simulink model "Final_PAPER2_wtdelay_LQR"  (R2024b)
settings: Solver=ode23  StartTime=0.0  StopTime=6  RelTol=1e-3
undefined symbols (not defined in the file): Q, R, sigbuilder_block
libraries: simulink_extras x4, simulink x1
settings Model: Creator=HP  LastModifiedBy=shree
settings OptimizationCC: ReuseModelBlockBuffer=off
settings RTWCC: GPUComputeCapability=3.5

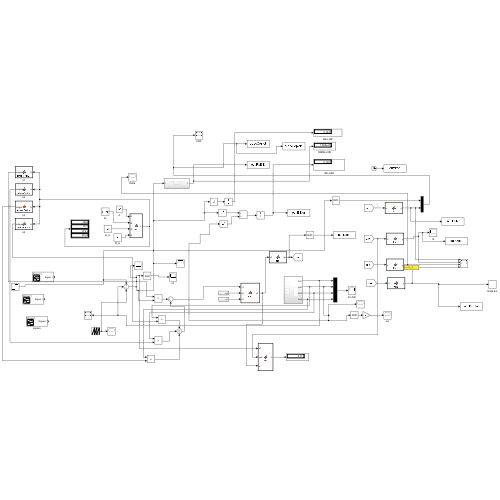
[thumbnail: Simulink's stored preview of the top-level diagram]
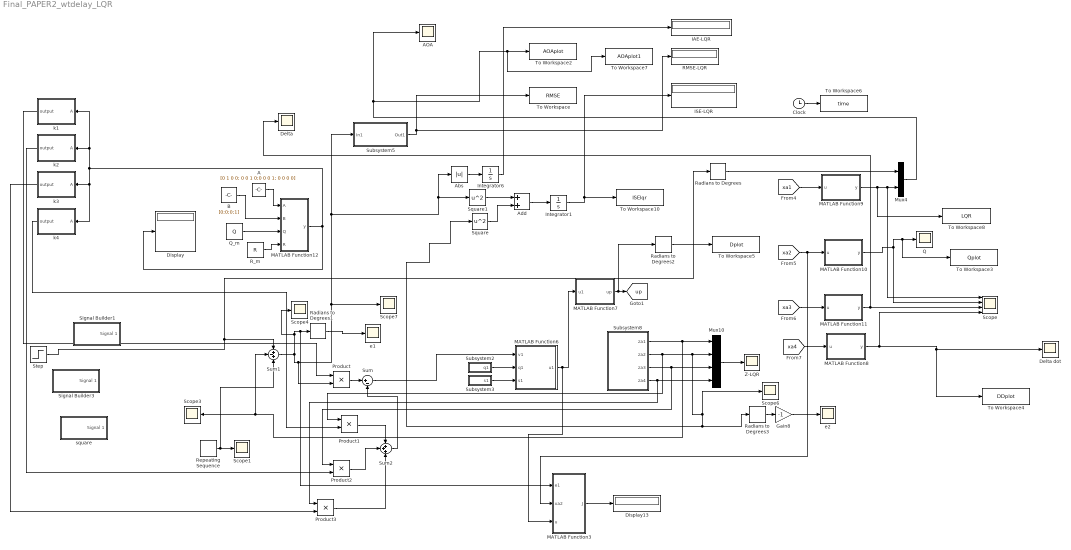
== system Final_PAPER2_wtdelay_LQR ==
  A : Constant  Value=[0 1 0 0; 0 0 1 0;0 0 0 1; 0 0 0 0]
  AOA : Scope
  Abs : Abs  SaturateOnIntegerOverflow=off
  Add : Sum
  B : Constant  Value=[0;0;0;1]
  Clock : Clock
      settings: Decimation=6
  Delta : Scope
  Delta dot : Scope
  Display : Display
  Display13 : Display
  Gain8 : Gain  Gain=-1
  IAE-LQR : Display
  ISE-LQR : Display
  Integrator1 : Integrator
  Integrator6 : Integrator
  MATLAB Function10 : MATLAB Function  TreatAsAtomicUnit=on
  MATLAB Function11 : MATLAB Function  TreatAsAtomicUnit=on
  MATLAB Function12 : MATLAB Function  TreatAsAtomicUnit=on
  MATLAB Function3 : MATLAB Function  TreatAsAtomicUnit=on
  MATLAB Function6 : MATLAB Function  TreatAsAtomicUnit=on
  MATLAB Function7 : MATLAB Function  TreatAsAtomicUnit=on
  MATLAB Function8 : MATLAB Function  TreatAsAtomicUnit=on
  MATLAB Function9 : MATLAB Function  TreatAsAtomicUnit=on
  Mux10 : Mux
  Mux4 : Mux  Inputs=2
  Product{,1..3} (4 alike) : Product
  Q : Scope
  Q_m : Constant  Value=Q
  RMSE-LQR : Display
  R_m : Constant  Value=R
  Radians to Degrees{,1..3} (4 alike) : simulink_extras/Transformations/Radians to Degrees
  Repeating Sequence : simulink/Sources/Repeating Sequence  rep_seq_t=t  rep_seq_y=u_combined
  Scope : Scope  NumInputPorts=4
  Scope{1,3..4,6..7} (5 alike) : Scope
  Signal Builder1 : Subsystem  Tag=STV Subsys  LoadFcn=sigbuilder_block('load');  StartFcn=sigbuilder_block('start');  StopFcn=sigbuilder_block('stop');  ClipboardFcn=sigbuilder_block('clipboard');  mask(Sigbuilder block){tuvar=[0:10]}
      mask help: Simulink:masks:SigbuilderBlock_MD
      mask init:
      | if ~strcmp(get_param(bdroot(gcbh),'SimulationStatus'),'stopped') tuvar = sigbuilder_block('maskInit'); end
      settings: CopyFcn=sigbuilder_block('copy');  DeleteFcn=sigbuilder_block('delete');  ModelCloseFcn=sigbuilder_block('modelClose');  PreSaveFcn=sigbuilder_block('preSave');  PauseFcn=sigbuilder_block('pause');  ContinueFcn=sigbuilder_block('continue');  NameChangeFcn=sigbuilder_block('namechange');  OpenFcn=sigbuilder_block('open',[5.4 -24.6 1141.2 477.6 ]);  CloseFcn=sigbuilder_block('close');
      mask Display: plot(0, 0, 100, 100,[2, 2, 32, 32, 2], [68, 8, 8, 68, 68],[32, 2], [38, 38], [32, 19, 2],[53, 60, 44], [32, 17, 17, 2],[16, 16, 31, 31]);txt = getActiveGroup(gcbh);text(2, 100, txt,'verticalAlignment', 'top');
  Signal Builder3 : Subsystem  Tag=STV Subsys  LoadFcn=sigbuilder_block('load');  StartFcn=sigbuilder_block('start');  StopFcn=sigbuilder_block('stop');  ClipboardFcn=sigbuilder_block('clipboard');  mask(Sigbuilder block){tuvar=[0:10]}
      mask help: Simulink:masks:SigbuilderBlock_MD
      mask init:
      | if ~strcmp(get_param(bdroot(gcbh),'SimulationStatus'),'stopped') tuvar = sigbuilder_block('maskInit'); end
      settings: CopyFcn=sigbuilder_block('copy');  DeleteFcn=sigbuilder_block('delete');  ModelCloseFcn=sigbuilder_block('modelClose');  PreSaveFcn=sigbuilder_block('preSave');  PauseFcn=sigbuilder_block('pause');  ContinueFcn=sigbuilder_block('continue');  NameChangeFcn=sigbuilder_block('namechange');  OpenFcn=sigbuilder_block('open',[5.4 -40.2 1141.2 515.4 ]);  CloseFcn=sigbuilder_block('close');
      mask Display: plot(0, 0, 100, 100,[2, 2, 32, 32, 2], [68, 8, 8, 68, 68],[32, 2], [38, 38], [32, 19, 2],[53, 60, 44], [32, 17, 17, 2],[16, 16, 31, 31]);txt = getActiveGroup(gcbh);text(2, 100, txt,'verticalAlignment', 'top');
  Square : Math  Operator=square
  Square1 : Math  Operator=square
  Step : Step  Time=0  After=0.2617795  SampleTime=0
  Subsystem2 : Subsystem
  Subsystem3 : Subsystem
  Subsystem5 : Subsystem
  Subsystem8 : Subsystem
  Sum : Sum  Inputs=|+-
  Sum1 : Sum  Inputs=+-+
  Sum2 : Sum  Inputs=+++
  To Workspace : ToWorkspace  VariableName=RMSE  SampleTime=-1
  To Workspace10 : ToWorkspace  VariableName=ISElqr  SampleTime=-1
  To Workspace2 : ToWorkspace  VariableName=AOAplot  SampleTime=-1
  To Workspace3 : ToWorkspace  VariableName=Qplot  SaveFormat=Timeseries  SampleTime=-1
  To Workspace4 : ToWorkspace  VariableName=DDplot  SaveFormat=Timeseries  SampleTime=-1
  To Workspace5 : ToWorkspace  VariableName=Dplot  SaveFormat=Timeseries  SampleTime=-1
  To Workspace6 : ToWorkspace  VariableName=time  SaveFormat=Timeseries  SampleTime=-1
  To Workspace7 : ToWorkspace  VariableName=AOAplot1  SampleTime=-1
  To Workspace8 : ToWorkspace  VariableName=LQR  SaveFormat=Timeseries  SampleTime=-1
  Z-LQR : Scope
  e1 : Scope
  e2 : Scope
  k1 : MATLAB Function  TreatAsAtomicUnit=on
  k2 : MATLAB Function  TreatAsAtomicUnit=on
  k3 : MATLAB Function  TreatAsAtomicUnit=on
  k4 : MATLAB Function  TreatAsAtomicUnit=on
  square : Subsystem  Tag=STV Subsys  LoadFcn=sigbuilder_block('load');  StartFcn=sigbuilder_block('start');  StopFcn=sigbuilder_block('stop');  ClipboardFcn=sigbuilder_block('clipboard');  mask(Sigbuilder block){tuvar=[0:10]}
      mask help: Simulink:masks:SigbuilderBlock_MD
      mask init:
      | if ~strcmp(get_param(bdroot(gcbh),'SimulationStatus'),'stopped') tuvar = sigbuilder_block('maskInit'); end
      settings: CopyFcn=sigbuilder_block('copy');  DeleteFcn=sigbuilder_block('delete');  ModelCloseFcn=sigbuilder_block('modelClose');  PreSaveFcn=sigbuilder_block('preSave');  PauseFcn=sigbuilder_block('pause');  ContinueFcn=sigbuilder_block('continue');  NameChangeFcn=sigbuilder_block('namechange');  OpenFcn=sigbuilder_block('open',[5.4 36 1141.2 516.6 ]);  CloseFcn=sigbuilder_block('close');
      mask Display: plot(0, 0, 100, 100,[2, 2, 32, 32, 2], [68, 8, 8, 68, 68],[32, 2], [38, 38], [32, 19, 2],[53, 60, 44], [32, 17, 17, 2],[16, 16, 31, 31]);txt = getActiveGroup(gcbh);text(2, 100, txt,'verticalAlignment', 'top');
  tag scope: up=global
  wires:
  [xa4] -> MATLAB Function8/1(u)
  Subsystem2/1(q1) -> MATLAB Function6/2(q1)
  Subsystem3/1(s1) -> MATLAB Function6/3(s1)
  MATLAB Function6/1(u1) -> MATLAB Function3/3(u), MATLAB Function7/1(u1)
  [xa3] -> MATLAB Function11/1(u)
  [xa2] -> MATLAB Function3/2(xa2), MATLAB Function10/1(u)
  MATLAB Function10/1(y) -> Scope/2, Q/1, To Workspace3/1
  MATLAB Function11/1(y) -> Delta/1, Scope/3
  [xa1] -> MATLAB Function9/1(u)
  Mux4/1 -> AOA/1, To Workspace7/1, To Workspace2/1
  Integrator1/1 -> To Workspace10/1, ISE-LQR/1
  Subsystem5/1(Out1) -> To Workspace/1, RMSE-LQR/1
  Sum1/1 -> Scope4/1, MATLAB Function3/1(e1), Radians to Degrees1/1, Product/2, Scope7/1, Square1/1, Abs/1, Subsystem5/1(In1)
  Abs/1 -> Integrator6/1
  Integrator6/1 -> IAE-LQR/1
  MATLAB Function7/1(up) -> Radians to Degrees2/1, [up]
  Mux10/1 -> Z-LQR/1
  Subsystem8/4(za4) -> Product3/1, Mux10/4
  Subsystem8/3(za3) -> Product2/1, Mux10/3
  Subsystem8/1(za1) -> Sum1/2, Scope3/1, Mux10/1
  MATLAB Function9/1(y) -> To Workspace8/1, Scope/1, Mux4/2
  MATLAB Function8/1(y) -> Scope/4, Delta dot/1, To Workspace4/1
  Radians to Degrees/1 -> Mux4/1
  Clock/1 -> To Workspace6/1
  Radians to Degrees1/1 -> e1/1
  Radians to Degrees2/1 -> To Workspace5/1
  Subsystem8/2(za2) -> Product1/1, Scope6/1, Radians to Degrees3/1, Square/1, Mux10/2
  Radians to Degrees3/1 -> Gain8/1
  Gain8/1 -> e2/1
  Add/1 -> Integrator1/1
  Square/1 -> Add/2
  Square1/1 -> Add/1
  MATLAB Function3/1(J) -> Display13/1
  Sum2/1 -> Sum/2
  Sum/1 -> MATLAB Function6/1(v1)
  Step/1 -> Radians to Degrees/1, Sum1/1
  MATLAB Function12/1(y) -> k1/1(A), k2/1(A), k4/1(A), k3/1(A), Display/1
  B/1 -> MATLAB Function12/2(B)
  A/1 -> MATLAB Function12/1(A)
  k1/1(output) -> Product/1
  Product/1 -> Sum/1
  k4/1(output) -> Product1/2
  Product1/1 -> Sum2/1
  k2/1(output) -> Product2/2
  Product2/1 -> Sum2/2
  k3/1(output) -> Product3/2
  Product3/1 -> Sum2/3
  Q_m/1 -> MATLAB Function12/3(Q)
  R_m/1 -> MATLAB Function12/4(R)
  Repeating Sequence/1 -> Sum1/3, Scope1/1

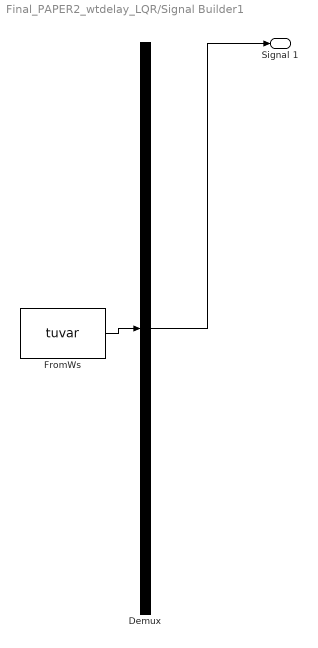
== system Final_PAPER2_wtdelay_LQR/Signal Builder1 ==
  Demux : Demux  Tag=STV Demux  Outputs=1
      settings: DisplayOption=none
  FromWs : FromWorkspace  Tag=STV FromWs  VariableName=tuvar
      SigBuilderData=|
      | common.afterFinalStr = 'Extrapolate'
      | common.sampleTime = 0
      | dataSet.timeRange = [0 10]
      | dataSet.name = 'Group 1'
      | sbobj.Groups.Name = 'Group 1'
      | sbobj.Groups.Signals.Name = 'Signal 1'
      | sbobj.Groups.Signals.XData = [0 2 2 4 4 6 6 8 8 10]
      | sbobj.Groups.Signals.YData = [-0.176 -0.176 0.176 0.176 -0.176 -0.176 0.176 0.176 -0.176 -0.176]
  Signal 1 : Outport  Tag=STV Outport
  wires:
  Demux/1 -> Signal 1/1
  FromWs/1 -> Demux/1

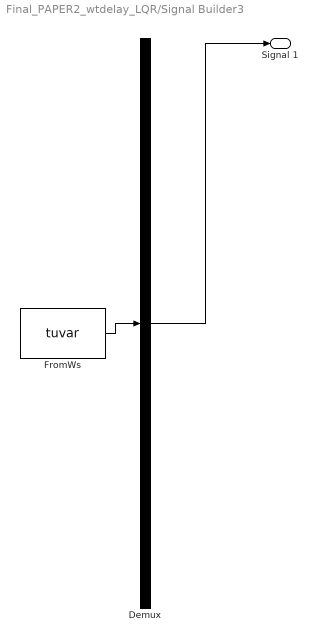
== system Final_PAPER2_wtdelay_LQR/Signal Builder3 ==
  Demux : Demux  Tag=STV Demux  Outputs=1
      settings: DisplayOption=none
  FromWs : FromWorkspace  Tag=STV FromWs  VariableName=tuvar
      SigBuilderData=|
      | common.afterFinalStr = 'Extrapolate'
      | common.sampleTime = 0
      | dataSet.timeRange = [0 6]
      | dataSet.name = 'Group 1'
      | sbobj.Groups.Name = 'Group 1'
      | sbobj.Groups.Signals.Name = 'Signal 1'
      | sbobj.Groups.Signals.XData = [0 2 2 4 4 6]
      | sbobj.Groups.Signals.YData = [0.261799 0.261799 -0.261799 -0.261799 0.261799 0.261799]
      | sbobj.Groups.TimeRange = [0 6]
  Signal 1 : Outport  Tag=STV Outport
  wires:
  Demux/1 -> Signal 1/1
  FromWs/1 -> Demux/1

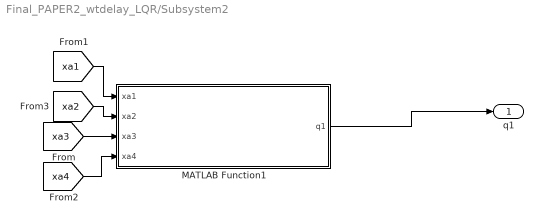
== system Final_PAPER2_wtdelay_LQR/Subsystem2 ==
  MATLAB Function1 : MATLAB Function  TreatAsAtomicUnit=on
  q1 : Outport
  wires:
  [xa2] -> MATLAB Function1/2(xa2)
  [xa1] -> MATLAB Function1/1(xa1)
  MATLAB Function1/1(q1) -> q1/1
  [xa3] -> MATLAB Function1/3(xa3)
  [xa4] -> MATLAB Function1/4(xa4)

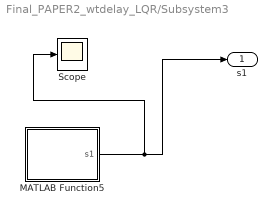
== system Final_PAPER2_wtdelay_LQR/Subsystem3 ==
  MATLAB Function5 : MATLAB Function  TreatAsAtomicUnit=on
  Scope : Scope
  s1 : Outport
  wires:
  MATLAB Function5/1(s1) -> Scope/1, s1/1

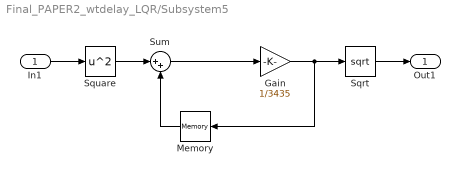
== system Final_PAPER2_wtdelay_LQR/Subsystem5 ==
  In1 : Inport
  Gain : Gain  Gain=1/3435
  Memory : Memory
  Sqrt : Sqrt
  Square : Math  Operator=square
  Sum : Sum  Inputs=|++
  Out1 : Outport
  wires:
  In1/1 -> Square/1
  Square/1 -> Sum/1
  Memory/1 -> Sum/2
  Sum/1 -> Gain/1
  Gain/1 -> Sqrt/1, Memory/1
  Sqrt/1 -> Out1/1

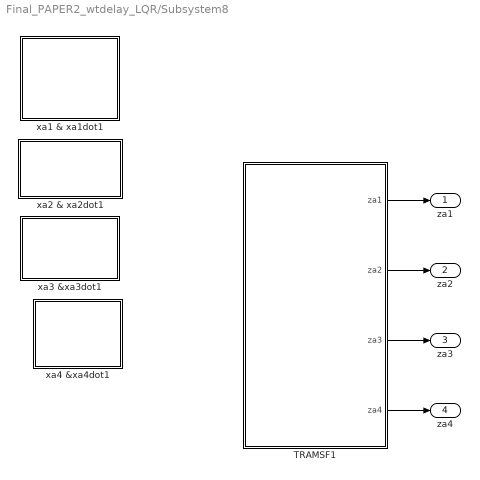
== system Final_PAPER2_wtdelay_LQR/Subsystem8 ==
  " xa3 &xa3dot1" : Subsystem
  TRAMSF1 : Subsystem
  xa1 & xa1dot1 : Subsystem
  xa2 & xa2dot1 : Subsystem
  xa4 &xa4dot1 : Subsystem
  za1 : Outport
  za2 : Outport  Port=2
  za3 : Outport  Port=3
  za4 : Outport  Port=4
  wires:
  TRAMSF1/1(za1) -> za1/1
  TRAMSF1/3(za3) -> za3/1
  TRAMSF1/2(za2) -> za2/1
  TRAMSF1/4(za4) -> za4/1

== system Final_PAPER2_wtdelay_LQR/square ==
  Demux : Demux  Tag=STV Demux  Outputs=1
      settings: DisplayOption=none
  FromWs : FromWorkspace  Tag=STV FromWs  VariableName=tuvar
      SigBuilderData=|
      | common.afterFinalStr = 'Extrapolate'
      | common.sampleTime = 0
      | dataSet.timeRange = [0 10]
      | dataSet.name = 'Group 1'
      | sbobj.Groups.Name = 'Group 1'
      | sbobj.Groups.Signals.Name = 'Signal 1'
      | sbobj.Groups.Signals.XData = [0 2 2 4 4 10]
      | sbobj.Groups.Signals.YData = [0.2617 0.2617 -0.176 -0.176 0.176 0.176]
  Signal 1 : Outport  Tag=STV Outport
  wires:
  Demux/1 -> Signal 1/1
  FromWs/1 -> Demux/1

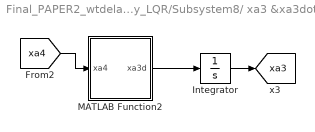
== system Final_PAPER2_wtdelay_LQR/Subsystem8/ xa3 &xa3dot1 ==
  Integrator : Integrator
  MATLAB Function2 : MATLAB Function  TreatAsAtomicUnit=on
  tag scope: xa3=global
  wires:
  Integrator/1 -> [xa3]
  [xa4] -> MATLAB Function2/1(xa4)
  MATLAB Function2/1(xa3d) -> Integrator/1

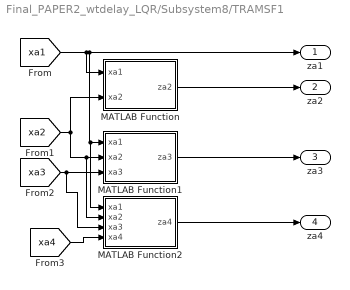
== system Final_PAPER2_wtdelay_LQR/Subsystem8/TRAMSF1 ==
  MATLAB Function : MATLAB Function  TreatAsAtomicUnit=on
  MATLAB Function1 : MATLAB Function  TreatAsAtomicUnit=on
  MATLAB Function2 : MATLAB Function  TreatAsAtomicUnit=on
  za1 : Outport
  za2 : Outport  Port=2
  za3 : Outport  Port=3
  za4 : Outport  Port=4
  wires:
  [xa1] -> MATLAB Function2/1(xa1), MATLAB Function1/1(xa1), za1/1, MATLAB Function/1(xa1)
  [xa2] -> MATLAB Function2/2(xa2), MATLAB Function1/2(xa2), MATLAB Function/2(xa2)
  MATLAB Function/1(za2) -> za2/1
  [xa3] -> MATLAB Function2/3(xa3), MATLAB Function1/3(xa3)
  MATLAB Function1/1(za3) -> za3/1
  [xa4] -> MATLAB Function2/4(xa4)
  MATLAB Function2/1(za4) -> za4/1

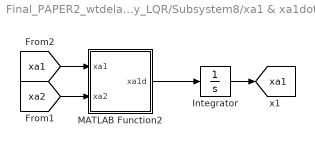
== system Final_PAPER2_wtdelay_LQR/Subsystem8/xa1 & xa1dot1 ==
  Integrator : Integrator
  MATLAB Function2 : MATLAB Function  TreatAsAtomicUnit=on
  tag scope: xa1=global
  wires:
  Integrator/1 -> [xa1]
  [xa1] -> MATLAB Function2/1(xa1)
  MATLAB Function2/1(xa1d) -> Integrator/1
  [xa2] -> MATLAB Function2/2(xa2)

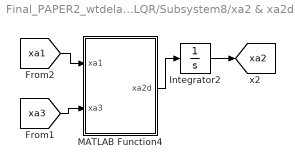
== system Final_PAPER2_wtdelay_LQR/Subsystem8/xa2 & xa2dot1 ==
  Integrator2 : Integrator
  MATLAB Function4 : MATLAB Function  TreatAsAtomicUnit=on
  tag scope: xa2=global
  wires:
  MATLAB Function4/1(xa2d) -> Integrator2/1
  Integrator2/1 -> [xa2]
  [xa3] -> MATLAB Function4/2(xa3)
  [xa1] -> MATLAB Function4/1(xa1)

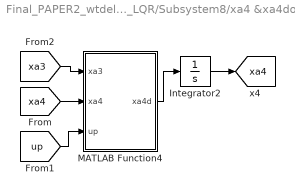
== system Final_PAPER2_wtdelay_LQR/Subsystem8/xa4 &xa4dot1 ==
  Integrator2 : Integrator
  MATLAB Function4 : MATLAB Function  TreatAsAtomicUnit=on
  tag scope: xa4=global
  wires:
  MATLAB Function4/1(xa4d) -> Integrator2/1
  Integrator2/1 -> [xa4]
  [xa3] -> MATLAB Function4/1(xa3)
  [up] -> MATLAB Function4/3(up)
  [xa4] -> MATLAB Function4/2(xa4)

== matlab function Final_PAPER2_wtdelay_LQR/MATLAB Function9 ==
  data: u input; y output
function y = fcn(u)

y = u*57.32;

== matlab function Final_PAPER2_wtdelay_LQR/Subsystem2/MATLAB Function1 ==
  data: q1 output; xa1 input; xa2 input; xa3 input; xa4 input
function q1 = fcn(xa1,xa2,xa3,xa4)
an=0.000103;
bn=-0.00945;
cn=-0.1696;
dn=-0.034;
am=0.000215;
bm=-0.0195;
cm=0.051;
dm=-0.206;
k=57.3248;
Kq=1.23202439;
Ka=0.020691432;
M=2.5;
wa=50;
zt = 1.4;
q1=dm*k*Kq*M^2*(-wa^2*xa3-wa*xa4*zt) + dm*k*Kq*M^2*xa4*(Ka*M*cos(xa1)*(cn*k*(2-M/3)+ 3*an*k^3*xa1^2+2*bn*k^2*abs(xa1))-Ka*M*(cn*k*(2-M/3)*xa1+an*k^3*xa1^3+bn*k^2*xa1*abs(xa1))*sin(xa1))+Kq*M^2*(cm*k*(-7 + (8*M)/3)*xa1 + am*k^3*xa1^3 + dm*k*xa3 + bm*k^2*xa1*abs(xa1))*(Kq*M^2*(cm*k*(-7 + (8*M)/3) +3*am*k^3*xa1^2 +2* bm*k^2*abs(xa1)) + 2*(xa2 + Ka*M*cos(xa1)*(cn*k*(2-M/3)*xa1 + an*k^3*xa1^3 +bn*k^2*xa1*abs(xa1)))*(Ka*M*cos(xa1)*(6*an*k^3*xa1 - bn*k^2*sign(xa1) + 3*bn*k^2*sign(xa1)) - Ka*M*cos(xa1)*(cn*k*(2-M/3)*xa1 + an*k^3*xa1^3 + bn*k^2*xa1*abs(xa1)) - 2*Ka*M*(cn*k*(2-M/3) + 3*an*k^3*xa1^2 + 2*bn*k^2*abs(xa1))*sin(xa1)) + (Ka*M*cos(xa1)*(cn*k*(2-M/3) + 3*an*k^3*xa1^2 + 2*bn*k^2*abs(xa1)) - Ka*M*(cn*k*(2-M/3)*xa1 + an*k^3*xa1^3 + bn*k^2*xa1*abs(xa1))*sin(xa1))^2) + (xa2 + Ka*M*cos(xa1)*(cn*k*(2-M/3)*xa1 + an*k^3*xa1^3 + bn*k^2*xa1*abs(xa1)))*(Kq*M^2*(cm*k*(-7 + (8*M)/3)*xa1 + am*k^3*xa1^3 + dm*k*xa3 + bm*k^2*xa1*abs(xa1))*(Ka*M*cos(xa1)*(6*an*k^3*xa1 - bn*k^2*sign(xa1) + 3*bn*k^2*sign(xa1))-Ka*M*cos(xa1)*(cn*k*(2-M/3)*xa1+an*k^3*xa1^3+bn*k^2*xa1*abs(xa1))-2*Ka*M*(cn*k*(2-M/3)+3*an*k^3*xa1^2+2*bn*k^2*abs(xa1))*sin(xa1))+ Kq*M^2*(cm*k*(-7+(8*M)/3)+3*am*k^3*xa1^2+2*bm*k^2*abs(xa1))*(Ka*M*cos(xa1)*(cn*k*(2-M/3)+3*an*k^3*xa1^2+2*bn*k^2*abs(xa1)) - Ka*M*(cn*k*(2-M/3)*xa1+an*k^3*xa1^3+bn*k^2*xa1*abs(xa1))*sin(xa1))+(Ka*M*cos(xa1)*(cn*k*(2-M/3)+3*an*k^3*xa1^2+2*bn*k^2*abs(xa1)) - Ka*M*(cn*k*(2-M/3)*xa1+an*k^3*xa1^3+bn*k^2*xa1*abs(xa1))*sin(xa1))*(Kq*M^2*(cm*k*(-7+(8*M)/3)+3*am*k^3*xa1^2+2*bm*k^2*abs(xa1))+(xa2 + Ka*M*cos(xa1)*(cn*k*(2-M/3)*xa1+an*k^3*xa1^3+bn*k^2*xa1*abs(xa1)))*(Ka*M*cos(xa1)*(6*an*k^3*xa1 - bn*k^2*sign(xa1) + 3*bn*k^2*sign(xa1))-Ka*M*cos(xa1)*(cn*k*(2-M/3)*xa1+an*k^3*xa1^3+bn*k^2*xa1*abs(xa1))-2*Ka*M*(cn*k*(2-M/3) + 3*an*k^3*xa1^2 + 2*bn*k^2*abs(xa1))*sin(xa1))+(Ka*M*cos(xa1)*(cn*k*(2-M/3) + 3*an*k^3*xa1^2 + 2*bn*k^2*abs(xa1)) - Ka*M*(cn*k*(2-M/3)*xa1 + an*k^3*xa1^3 + bn*k^2*xa1*abs(xa1))*sin(xa1))^2)+(xa2 + Ka*M*cos(xa1)*(cn*k*(2-M/3)*xa1 + an*k^3*xa1^3 +bn*k^2*xa1*abs(xa1)))*(Kq*M^2*(6*am*k^3*xa1-bm*k^2*sign(xa1)+3*bm*k^2*sign(xa1)) + 3*(Ka*M*cos(xa1)*(6*an*k^3*xa1-bn*k^2*sign(xa1)+3*bn*k^2*sign(xa1)) - Ka*M*cos(xa1)*(cn*k*(2-M/3)*xa1+an*k^3*xa1^3+bn*k^2*xa1*abs(xa1)) - 2*Ka*M*(cn*k*(2-M/3)+3*an*k^3*xa1^2+2*bn*k^2*abs(xa1))*sin(xa1))*(Ka*M*cos(xa1)*(cn*k*(2-M/3)+3*an*k^3*xa1^2+2*bn*k^2*abs(xa1)) - Ka*M*(cn*k*(2-M/3)*xa1+an*k^3*xa1^3+bn*k^2*xa1*abs(xa1))*sin(xa1))+(xa2 + Ka*M*cos(xa1)*(cn*k*(2-M/3)*xa1+an*k^3*xa1^3+bn*k^2*xa1*abs(xa1)))*(Ka*M*cos(xa1)*6*an*k^3-3*Ka*M*cos(xa1)*(cn*k*(2-M/3)+3*an*k^3*xa1^2+2*bn*k^2*abs(xa1))-3*Ka*M*(6*an*k^3*xa1-bn*k^2*sign(xa1)+3*bn*k^2*sign(xa1))*sin(xa1)+Ka*M*(cn*k*(2-M/3)*xa1+an*k^3*xa1^3+bn*k^2*xa1*abs(xa1))*sin(xa1))));

== matlab function Final_PAPER2_wtdelay_LQR/Subsystem3/MATLAB Function5 ==
  data: s1 output
function s1 = fcn()
an=0.000103;
bn=-0.00945;
cn=-0.1696;
dn=-0.034;
am=0.000215;
bm=-0.0195;
cm=0.051;
dm=-0.206;
k=57.32;
wa=50;
Kq=1.23202439;
em=-0.03000221;
M=2.5;
s1=Kq*dm*k*wa^2*M^2;

== matlab function Final_PAPER2_wtdelay_LQR/Subsystem8/TRAMSF1/MATLAB Function ==
  data: xa1 input; za2 output; xa2 input
function za2 = fcn(xa1,xa2)
an=0.000103;
bn=-0.00945;
cn=-0.1696;
dn=-0.034;
am=0.000215;
bm=-0.0195;
cm=0.051;
dm=-0.206;
k=57.3248;
em=-0.03000221;
Kq=1.23202439;
Ka=0.020691432;
M=2.5;
wa=50;
za2 = xa2 + k*Ka*M*xa1*cos(xa1) * (-1/3*cn*(-6+M) + an*k^2*xa1^2 + bn*k*abs(xa1));

== matlab function Final_PAPER2_wtdelay_LQR/Subsystem8/TRAMSF1/MATLAB Function1 ==
  data: xa1 input; za3 output; xa2 input; xa3 input
function za3 = fcn(xa1,xa2,xa3)
an=0.000103;
bn=-0.00945;
cn=-0.1696;
dn=-0.034;
am=0.000215;
bm=-0.0195;
cm=0.051;
dm=-0.206;
k=57.3248;
em=-0.03000221;
Kq=1.23202439;
Ka=0.020691432;
M=2.5;
wa=50;
za3=M*(k*Kq*M*(cm*(-7 + (8*M)/3)*xa1 + am*k^2*xa1^3 + dm*xa3 + bm*k*xa1*abs(xa1)) + Ka*(xa2 + k*Ka*M*xa1*cos(xa1)*(-(1/3)*cn*(-6 + M) + an*k^2*xa1^2 + bn*k*abs(xa1)))*(k*cos(xa1)*(-(1/3)*cn*(-6 + M) + 3*an*k^2*xa1^2 + 2*bn*k*abs(xa1)) + (1/3)*k*xa1*(cn*(-6 + M) - 3*an*k^2*xa1^2 - 3*bn*k*abs(xa1))*sin(xa1)));

== matlab function Final_PAPER2_wtdelay_LQR/Subsystem8/TRAMSF1/MATLAB Function2 ==
  data: xa1 input; za4 output; xa2 input; xa3 input; xa4 input
function za4 = fcn(xa1,xa2,xa3,xa4)
an=0.000103;
bn=-0.00945;
cn=-0.1696;
dn=-0.034;
am=0.000215;
bm=-0.0195;
cm=0.051;
dm=-0.206;
k=57.3248;
em=-0.03000221;
Kq=1.23202439;
Ka=0.020691432;
M=2.5;
wa=50;
za4 = dm*k*Kq*M^2*xa4 + Kq*M^2*(cm*k*(-7 + (8*M)/3)*xa1 + am*k^3*xa1^3 + dm*k*xa3 + bm*k^2*xa1*abs(xa1))*(Ka*M*cos(xa1)*(cn*k*(2 - M/3) + 3*an*k^3*xa1^2 + bn*k^2*abs(xa1) + bn*k^2*abs(xa1))-Ka*M*(cn*k*(2 - M/3)*xa1 + an*k^3*xa1^3 + bn*k^2*xa1*abs(xa1))*sin(xa1)) + (xa2 + Ka*M*cos(xa1)*(cn*k*(2 - M/3)*xa1 + an*k^3*xa1^3 + bn*k^2*xa1*abs(xa1)))*(Kq*M^2*(cm*k*(-7 + (8*M)/3) + 3*am*k^3*xa1^2 + bm*k^2*abs(xa1) + bm*k^2*abs(xa1))+(xa2 + Ka*M*cos(xa1)*(cn*k*(2 - M/3)*xa1 + an*k^3*xa1^3 + bn*k^2*xa1*abs(xa1)))*(Ka*M*cos(xa1)*(6*an*k^3*xa1 - (bn*k^2*sign(xa1)) + 3*bn*k^2*sign(xa1))-Ka*M*cos(xa1)*(cn*k*(2 - M/3)*xa1 + an*k^3*xa1^3 + bn*k^2*xa1*abs(xa1))-2*Ka*M*(cn*k*(2 - M/3) + 3*an*k^3*xa1^2 + bn*k^2*abs(xa1) + bn*k^2*abs(xa1))*sin(xa1))+(Ka*M*cos(xa1)*(cn*k*(2 - M/3) + 3*an*k^3*xa1^2 + bn*k^2*abs(xa1) + bn*k^2*abs(xa1))-Ka*M*(cn*k*(2 - M/3)*xa1 + an*k^3*xa1^3 + bn*k^2*xa1*abs(xa1))*sin(xa1))^2);

== matlab function Final_PAPER2_wtdelay_LQR/k1 ==
  data: A input; output output
function output = extractValue(A)
    output = A(1, 1); 
end

== matlab function Final_PAPER2_wtdelay_LQR/Subsystem8/xa1 & xa1dot1/MATLAB Function2 ==
  data: xa1 input; xa1d output; xa2 input
function xa1d = fcn(xa1,xa2)
an=0.000103;
bn=-0.00945;
cn=-0.1696;
dn=-0.034;
am=0.000215;
bm=-0.0195;
cm=0.051;
dm=-0.206;
k=180/pi;
Ka=0.020691432;
Kq=1.23202439;
em=-0.03000221;
M=2.5;
wa=50;
xa1d=Ka*M*(an*xa1^3*k^3 + bn*xa1*abs(xa1)*k^2 + cn*(2 - (M/3))*xa1*k)*cos(xa1) + xa2;

== matlab function Final_PAPER2_wtdelay_LQR/Subsystem8/xa2 & xa2dot1/MATLAB Function4 ==
  data: xa1 input; xa2d output; xa3 input
function xa2d = fcn(xa1,xa3)
an=0.000103;
bn=-0.00945;
cn=-0.1696;
dn=-0.034;
am=0.000215;
bm=-0.0195;
cm=0.051;
dm=-0.206;
k=57.3248;
Ka=0.020691432;
Kq=1.23202439;
em=-0.03000221;
M=2.5;
wa=50;
xa2d=Kq*M^2*(am*xa1^3*k^3 + bm*xa1*abs(xa1)*k^2 + cm*(-7 + (8*M/3))*xa1*k + dm*k*xa3);

== matlab function Final_PAPER2_wtdelay_LQR/Subsystem8/xa4 &xa4dot1/MATLAB Function4 ==
  data: xa3 input; xa4 input; xa4d output; up input
function xa4d = fcn(xa3,xa4,up)
an=0.000103;
bn=-0.00945;
cn=-0.1696;
dn=-0.034;
am=0.000215;
bm=-0.0195;
cm=0.051;
dm=-0.206;
k=57.3248;
em=-0.03000221;
M=2.5;
wa=50;
zt=1.4
xa4d= -wa^2*xa3 -zt*wa*xa4 + wa^2*up;

== matlab function Final_PAPER2_wtdelay_LQR/MATLAB Function3 ==
  data: e1 input; J output; xa2 input; u input
function  J = fcn(e1,xa2,u)

J=e1*e1+xa2*xa2+u*u;

== matlab function Final_PAPER2_wtdelay_LQR/MATLAB Function12 ==
  data: A input; y output; B input; Q input; R input
function y = fcn(A,B,Q,R)
y = zeros(1,4);
coder.extrinsic('lqr');
y = lqr(A,B,Q,R);

== matlab function Final_PAPER2_wtdelay_LQR/Subsystem8/ xa3 &xa3dot1/MATLAB Function2 ==
  data: xa4 input; xa3d output
function xa3d = fcn(xa4)
xa3d=xa4;

== matlab function Final_PAPER2_wtdelay_LQR/k4 ==
  data: A input; output output
function output = extractValue(A)
    output = A(1, 2); 
end

== matlab function Final_PAPER2_wtdelay_LQR/MATLAB Function10 ==
  data: u input; y output
function y = fcn(u)

y = u*57.32;

== matlab function Final_PAPER2_wtdelay_LQR/k2 ==
  data: A input; output output
function output = extractValue(A)
    output = A(1, 3); 
end

== matlab function Final_PAPER2_wtdelay_LQR/k3 ==
  data: A input; output output
function output = extractValue(A)
    output = A(1,4 ...
        ); 
end

== matlab function Final_PAPER2_wtdelay_LQR/MATLAB Function11 ==
  data: u input; y output
function y = fcn(u)

y = u*57.32;

== matlab function Final_PAPER2_wtdelay_LQR/MATLAB Function6 ==
  data: v1 input; u1 output; q1 input; s1 input
function u1 = fcn(v1,q1,s1)
u1 = (v1-q1)/s1;

== matlab function Final_PAPER2_wtdelay_LQR/MATLAB Function7 ==
  data: u1 input; up output
function up = fcn(u1)

up = u1;

== matlab function Final_PAPER2_wtdelay_LQR/MATLAB Function8 ==
  data: u input; y output
function y = fcn(u)

y = u*57.32;
